simulink model "pid_model"  (R2016b)
settings: Solver=ode4  StartTime=0.0  StopTime=1  FixedStep=0.02  RelTol=1e-3
values from neighbouring files (symbols this model uses):
  A0 = (sig(4)*rho(4)/(rho(1)+rho(2)))/base    [PID.m]
  A1 = (rho(4)/(rho(1)+rho(2))+rho(3)/(rho(1)+rho(2))*(sig(3)+sig(4)))/base    [PID.m]    (also in testLinearPara.m = (-(sig(1)+2*sig(2))*rho(4))/base)
  A2 = (rho(3)/(rho(1)+rho(2))-sig(3)-rho(3)/(rho(1)+rho(2))*(sig(1)+2*sig(2)+sig(4)/rho(3)))/base    [PID.m]    (also in testLinearPara.m = (-(sig(4)+(sig(1)+2*sig(2))*rho(3)))/base)
  A3 = (sig(1)+2*sig(2)-1/(rho(1)+rho(2)))/base    [PID.m]    (also in testLinearPara.m = (sig(3)-(sig(1)+2*sig(2))*rho(3))/base)
  Kd = (A3*(poles(1)+poles(2)+poles(3))+A2)*pi/180    [PID.m]
  Ki = (A3*(poles(1)*poles(2)*poles(3))+A0)*pi/180    [PID.m]
  Kp = (A1-A3*(poles(1)*poles(2)+poles(1)*poles(3)+poles(2)*poles(3)))*pi/180    [PID.m]
settings Model: Creator=Ernie  LastModifiedBy=Ernie

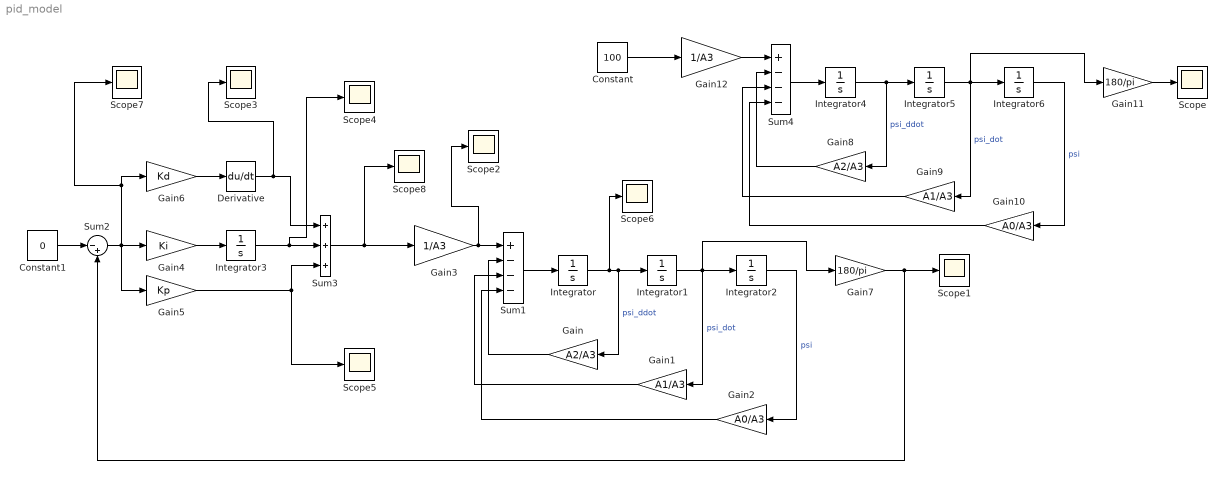
== system pid_model ==
  Constant : Constant  Value=100
  Constant1 : Constant  Value=0
  Derivative : Derivative
  Gain : Gain  Gain=A2/A3
  Gain1 : Gain  Gain=A1/A3
  Gain10 : Gain  Gain=A0/A3
  Gain11 : Gain  Gain=180/pi
  Gain12 : Gain  Gain=1/A3
  Gain2 : Gain  Gain=A0/A3
  Gain3 : Gain  Gain=1/A3
  Gain4 : Gain  Gain=Ki
  Gain5 : Gain  Gain=Kp
  Gain6 : Gain  Gain=Kd
  Gain7 : Gain  Gain=180/pi
  Gain8 : Gain  Gain=A2/A3
  Gain9 : Gain  Gain=A1/A3
  Integrator{,2..6} (6 alike) : Integrator
  Integrator1 : Integrator  InitialCondition=0.0843
  Scope{,1..8} (9 alike) : Scope
  Sum1 : Sum  Inputs=+---
  Sum2 : Sum  Inputs=|-+
  Sum3 : Sum  Inputs=+++
  Sum4 : Sum  Inputs=+---
  wires:
  Integrator/1 -> Scope6/1, Gain/1, Integrator1/1  "psi_ddot"
  Integrator1/1 -> Gain7/1, Gain1/1, Integrator2/1  "psi_dot"
  Sum1/1 -> Integrator/1
  Gain/1 -> Sum1/2
  Gain1/1 -> Sum1/3
  Integrator2/1 -> Gain2/1  "psi"
  Gain2/1 -> Sum1/4
  Gain3/1 -> Scope2/1, Sum1/1
  Constant1/1 -> Sum2/1
  Sum3/1 -> Scope8/1, Gain3/1
  Gain4/1 -> Integrator3/1
  Integrator3/1 -> Scope4/1, Sum3/2
  Gain5/1 -> Scope5/1, Sum3/3
  Derivative/1 -> Scope3/1, Sum3/1
  Gain6/1 -> Derivative/1
  Gain7/1 -> Sum2/2, Scope1/1
  Integrator4/1 -> Gain8/1, Integrator5/1  "psi_ddot"
  Integrator5/1 -> Gain11/1, Gain9/1, Integrator6/1  "psi_dot"
  Sum4/1 -> Integrator4/1
  Gain8/1 -> Sum4/2
  Gain9/1 -> Sum4/3
  Integrator6/1 -> Gain10/1  "psi"
  Gain10/1 -> Sum4/4
  Gain12/1 -> Sum4/1
  Constant/1 -> Gain12/1
  Gain11/1 -> Scope/1
  Sum2/1 -> Scope7/1, Gain6/1, Gain5/1, Gain4/1
